simulink model "problem1"  (R2020b)
settings: Solver=VariableStepAuto  StartTime=0.0  StopTime=10.0  RelTol=1e-3
settings Model: Creator=Shree  LastModifiedBy=Shree

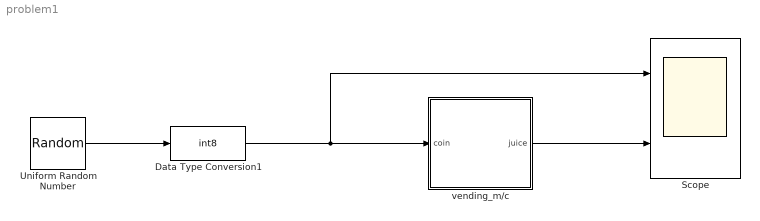
== system problem1 ==
  Data Type Conversion1 : DataTypeConversion  OutDataTypeStr=int8  RndMeth=Nearest  SaturateOnIntegerOverflow=on
  Scope : Scope  NumInputPorts=2
  Uniform Random Number : UniformRandomNumber  Minimum=0  Maximum=2  Seed=337  SampleTime=10
  vending_m/c : Stateflow chart  TreatAsAtomicUnit=on
  wires:
  vending_m/c/1(juice) -> Scope/2
  Uniform Random Number/1 -> Data Type Conversion1/1
  Data Type Conversion1/1 -> Scope/1, vending_m/c/1(coin)

== stateflow chart problem1/vending_m//c ==
  state got_0
  state got_dime
  state got_nickel
  (default) -> got_0
  got_0 -> got_dime [order 2] : [coin==2]{juice=0}
  got_dime -> got_0 [order 1] : [coin==1]{juice=1}
  got_0 -> got_nickel [order 1] : [coin==1]{juice=0}
  got_nickel -> got_0 [order 2] : [coin==2]{juice=1}
  got_nickel -> got_dime [order 1] : [coin==1]{juice=0}
  got_dime -> got_nickel [order 2] : [coin==2]{juice=1}
  data: coin input; juice output
